simulink subsystem "CONTROL_DETUMBLING"  (R2025b)
settings: Solver=VariableStepAuto  StartTime=0.0  StopTime=10.0  RelTol=1e-3
undefined symbols (not defined in the file): magUpdateFreq, mtqAllocationMatrix, mtqMagneticGain, mtqMaxMagDip, mtqResistance
settings Model: Creator=antoniohernandez-rodiciomateos  LastModifiedBy=antoniohernandez-rodiciomateos

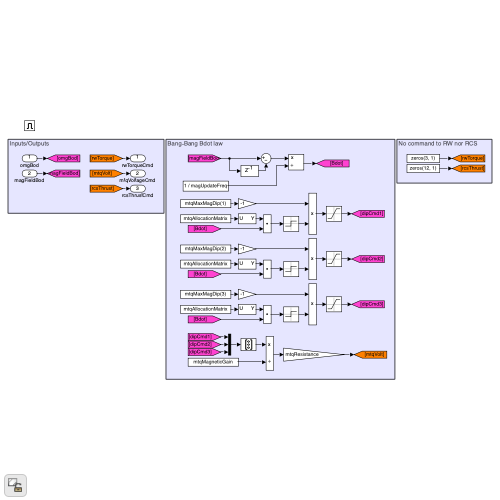
[thumbnail: Simulink's stored preview of the top-level diagram]
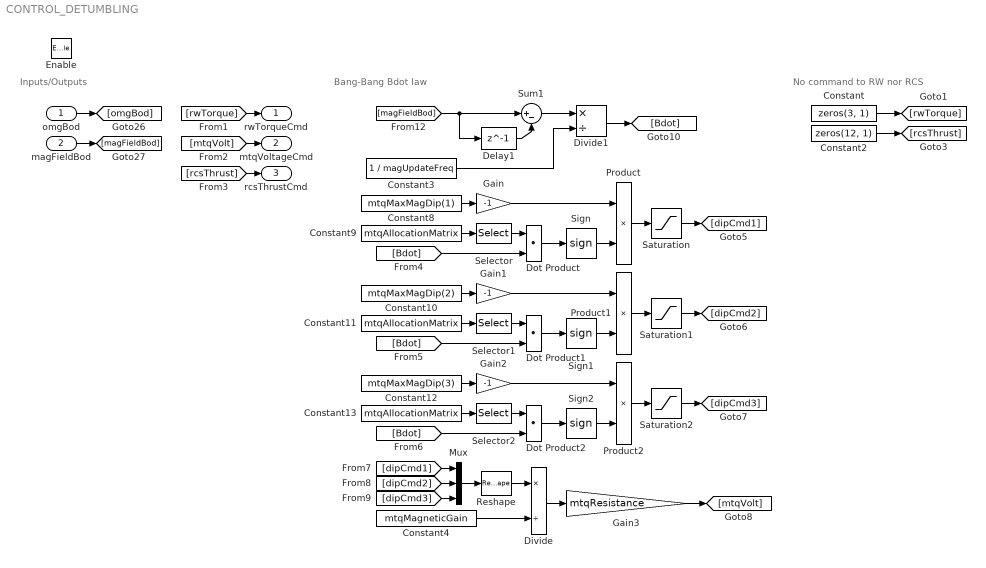
== system CONTROL_DETUMBLING ==
  note: Inputs/Outputs
  note: Bang-Bang Bdot law
  note: No command to RW nor RCS
  omgBod : Inport  OutDataTypeStr=double  PortDimensions=[3 1]
  magFieldBod : Inport  Port=2  OutDataTypeStr=double  PortDimensions=[3 1]
  Enable : EnablePort
  Constant : Constant  Value=zeros(3, 1)
  Constant10 : Constant  Value=mtqMaxMagDip(2)
  Constant11 : Constant  Value=mtqAllocationMatrix
  Constant12 : Constant  Value=mtqMaxMagDip(3)
  Constant13 : Constant  Value=mtqAllocationMatrix
  Constant2 : Constant  Value=zeros(12, 1)
  Constant3 : Constant  Value=1 / magUpdateFreq
  Constant4 : Constant  Value=mtqMagneticGain
  Constant8 : Constant  Value=mtqMaxMagDip(1)
  Constant9 : Constant  Value=mtqAllocationMatrix
  Delay1 : Delay  DelayLength=1  InitialCondition=zeros(3,1)
  Divide : Product  Inputs=*/
  Divide1 : Product  Inputs=*/
  Dot Product : DotProduct  OutDataTypeStr=Inherit: Inherit via internal rule
  Dot Product1 : DotProduct  OutDataTypeStr=Inherit: Inherit via internal rule
  Dot Product2 : DotProduct  OutDataTypeStr=Inherit: Inherit via internal rule
  Gain : Gain  Gain=-1
  Gain1 : Gain  Gain=-1
  Gain2 : Gain  Gain=-1
  Gain3 : Gain  Gain=mtqResistance
  Mux : Mux  Inputs=3
  Product : Product
  Product1 : Product
  Product2 : Product
  Reshape : Reshape  OutputDimensionality=Column vector (2-D)
  Saturation : Saturate  UpperLimit=mtqMaxMagDip(1)  LowerLimit=-1 * mtqMaxMagDip(1)
  Saturation1 : Saturate  UpperLimit=mtqMaxMagDip(2)  LowerLimit=-1 * mtqMaxMagDip(2)
  Saturation2 : Saturate  UpperLimit=mtqMaxMagDip(3)  LowerLimit=-1 * mtqMaxMagDip(1)
  Selector : Selector  NumberOfDimensions=2  InputPortWidth=3  IndexOptions=Index vector (dialog),Index vector (dialog)  Indices=[1 2 3],1  OutputSizes=1,1
  Selector1 : Selector  NumberOfDimensions=2  InputPortWidth=3  IndexOptions=Index vector (dialog),Index vector (dialog)  Indices=[1 2 3],2  OutputSizes=1,1
  Selector2 : Selector  NumberOfDimensions=2  InputPortWidth=3  IndexOptions=Index vector (dialog),Index vector (dialog)  Indices=[1 2 3],3  OutputSizes=1,1
  Sign : Signum
  Sign1 : Signum
  Sign2 : Signum
  Sum1 : Sum  Inputs=|+-
  rwTorqueCmd : Outport  OutDataTypeStr=double  PortDimensions=[3 1]
  mtqVoltageCmd : Outport  Port=2  OutDataTypeStr=double  PortDimensions=[3 1]
  rcsThrustCmd : Outport  Port=3  OutDataTypeStr=double  PortDimensions=[12 1]
  wires:
  omgBod/1 -> [omgBod]
  magFieldBod/1 -> [magFieldBod]
  [rwTorque] -> rwTorqueCmd/1
  [mtqVolt] -> mtqVoltageCmd/1
  [rcsThrust] -> rcsThrustCmd/1
  Constant/1 -> [rwTorque]
  Constant2/1 -> [rcsThrust]
  Constant8/1 -> Gain/1
  Constant9/1 -> Selector/1
  Selector/1 -> Dot Product/1
  [Bdot] -> Dot Product/2
  Dot Product/1 -> Sign/1
  Sign/1 -> Product/2
  Gain/1 -> Product/1
  Product/1 -> Saturation/1
  Saturation/1 -> [dipCmd1]
  Product1/1 -> Saturation1/1
  Constant11/1 -> Selector1/1
  Constant10/1 -> Gain1/1
  Dot Product1/1 -> Sign1/1
  Sign1/1 -> Product1/2
  Saturation1/1 -> [dipCmd2]
  Selector1/1 -> Dot Product1/1
  [Bdot] -> Dot Product1/2
  Gain1/1 -> Product1/1
  Product2/1 -> Saturation2/1
  Constant13/1 -> Selector2/1
  Constant12/1 -> Gain2/1
  Dot Product2/1 -> Sign2/1
  Sign2/1 -> Product2/2
  Saturation2/1 -> [dipCmd3]
  Selector2/1 -> Dot Product2/1
  [Bdot] -> Dot Product2/2
  Gain2/1 -> Product2/1
  [dipCmd3] -> Mux/3
  [dipCmd2] -> Mux/2
  [dipCmd1] -> Mux/1
  Mux/1 -> Reshape/1
  Reshape/1 -> Divide/1
  Constant4/1 -> Divide/2
  Divide/1 -> Gain3/1
  Gain3/1 -> [mtqVolt]
  [magFieldBod] -> Delay1/1, Sum1/1
  Delay1/1 -> Sum1/2
  Sum1/1 -> Divide1/1
  Constant3/1 -> Divide1/2
  Divide1/1 -> [Bdot]
